simulink model "gm_uz_pmsm_model_9ph_vnl"  (R2021a)
settings: Solver=FixedStepAuto  StartTime=0.0  StopTime=.5  RelTol=1e-3
PreLoadFcn:
  | uz_pmsm_model_init_parameter
undefined symbols (not defined in the file or in its folder): c, friction_coefficient, inertia, k_i_d, k_p_d, k_p_q, L_d, L_o1, L_o2, L_q, L_x1, L_x2, L_y1, L_y2, L_zero, polepair, psi_pm, R_1, static_friction_torque, ts
libraries: hdlmdlgenlib x220, hdlsllib x18, simulink x11, pid_lib x2
(part 2 of 4)

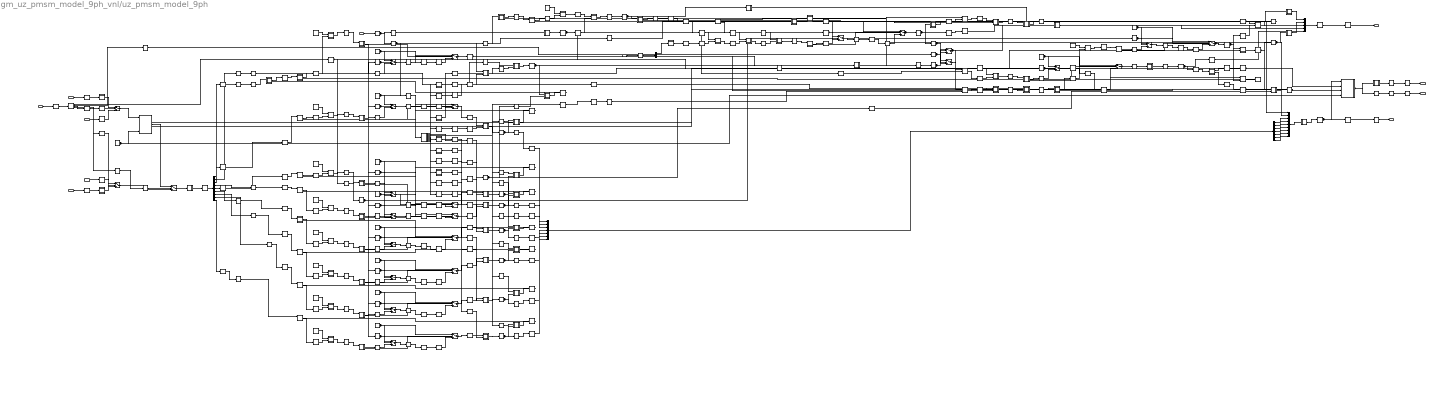
== system gm_uz_pmsm_model_9ph_vnl/uz_pmsm_model_9ph ==
  note: Input Processing
  note: o1 equation
  note: DQ equations
  note: o2 equation
  note: x1 equation
  note: y1 equation
  note: x2 equation
  note: y2 equation
  note: zero equation
  note: Output Processing
  Model_Parameter : Inport  SampleTime=1e-06
  Physical_Parameter : Inport  Port=2  SampleTime=1e-06
  inputs_general : Inport  Port=3  OutDataTypeStr=single  PortDimensions=[2]  SampleTime=1e-06
  input_voltages_dq : Inport  Port=4  OutDataTypeStr=single  PortDimensions=[9]  SampleTime=1e-06
  input_voltages_abc : Inport  Port=5  OutDataTypeStr=single  PortDimensions=[9]  SampleTime=1e-06
  u_dq_pl : Inport  Port=6  OutDataTypeStr=fixdt(1, 25, 12)  PortDimensions=[9]  SampleTime=1e-06
  u_abc_pl : Inport  Port=7  OutDataTypeStr=fixdt(1, 25, 12)  PortDimensions=[9]  SampleTime=1e-06
  Abs : Subsystem
      mask Display: disp('NFP\nabs');
  Abs_outbuff : hdlmdlgenlib/Buffer
      settings: SourceProductBaseCode=SL
  Add : Subsystem
      mask Display: disp('NFP\nadd');
  Add1 : Subsystem
      mask Display: disp('NFP\nadd');
  Add1_outbuff : hdlmdlgenlib/Buffer
      settings: SourceProductBaseCode=SL
  Add2 : Subsystem
      mask Display: disp('NFP\nadd');
  Add2_outbuff : hdlmdlgenlib/Buffer
      settings: SourceProductBaseCode=SL
  Add3 : Subsystem
      mask Display: disp('NFP\nadd');
  Add3_outbuff : hdlmdlgenlib/Buffer
      settings: SourceProductBaseCode=SL
  Add4 : Subsystem
      mask Display: disp('NFP\nadd');
  Add4_outbuff : hdlmdlgenlib/Buffer
      settings: SourceProductBaseCode=SL
  Add5 : Subsystem
      mask Display: disp('NFP\nadd');
  Add5_outbuff : hdlmdlgenlib/Buffer
      settings: SourceProductBaseCode=SL
  Add6 : Subsystem
      mask Display: disp('NFP\nadd');
  Add6_outbuff : hdlmdlgenlib/Buffer
      settings: SourceProductBaseCode=SL
  Add_outbuff : hdlmdlgenlib/Buffer
      settings: SourceProductBaseCode=SL
  Cos_to_sincos : Subsystem
      mask Display: disp('NFP\ntrig2');
  Cos_to_sincos_out1_buff : hdlmdlgenlib/Buffer
      settings: SourceProductBaseCode=SL
  Cos_to_sincos_out2_buff : hdlmdlgenlib/Buffer
      settings: SourceProductBaseCode=SL
  Data Type Conversion1 : Subsystem
      mask Display: disp('NFP\nconv');
  Data Type Conversion10 : Subsystem
      mask Display: disp('NFP\nconv');
  Data Type Conversion11 : Subsystem
      mask Display: disp('NFP\nconv');
  Data Type Conversion111 : Subsystem
      mask Display: disp('NFP\nconv');
  Data Type Conversion12 : Subsystem
      mask Display: disp('NFP\nconv');
  Data Type Conversion13 : Subsystem
      mask Display: disp('NFP\nconv');
  Data Type Conversion15 : Subsystem
      mask Display: disp('NFP\nconv');
  Data Type Conversion16 : Subsystem
      mask Display: disp('NFP\nconv');
  Data Type Conversion17 : Subsystem
      mask Display: disp('NFP\nconv');
  Data Type Conversion17_out1 : Delay  DelayLength=double(1)  InitialCondition=0  SampleTime=1e-08
  Data Type Conversion17_outbuff : hdlmdlgenlib/Buffer
      settings: SourceProductBaseCode=SL
  Data Type Conversion18 : Subsystem
      mask Display: disp('NFP\nconv');
  Data Type Conversion18_outbuff : hdlmdlgenlib/Buffer
      settings: SourceProductBaseCode=SL
  Data Type Conversion19 : Subsystem
      mask Display: disp('NFP\nconv');
  Data Type Conversion19_out1_0_wire : hdlmdlgenlib/Buffer
      settings: SourceProductBaseCode=SL
  Data Type Conversion19_out1_1_wire : hdlmdlgenlib/Buffer
      settings: SourceProductBaseCode=SL
  Data Type Conversion19_outbuff : hdlmdlgenlib/Buffer
      settings: SourceProductBaseCode=SL
  Data Type Conversion2 : Subsystem
      mask Display: disp('NFP\nconv');
  Data Type Conversion21 : Subsystem
      mask Display: disp('NFP\nconv');
  Data Type Conversion26 : Subsystem
      mask Display: disp('NFP\nconv');
  Data Type Conversion3 : Subsystem
      mask Display: disp('NFP\nconv');
  Data Type Conversion30 : Subsystem
      mask Display: disp('NFP\nconv');
  Data Type Conversion31 : Subsystem
      mask Display: disp('NFP\nconv');
  Data Type Conversion32 : Subsystem
      mask Display: disp('NFP\nconv');
  Data Type Conversion4 : Subsystem
      mask Display: disp('NFP\nconv');
  Data Type Conversion41 : Subsystem
      mask Display: disp('NFP\nconv');
  Data Type Conversion5 : Subsystem
      mask Display: disp('NFP\nconv');
  Data Type Conversion51 : Subsystem
      mask Display: disp('NFP\nconv');
  Data Type Conversion6 : Subsystem
      mask Display: disp('NFP\nconv');
  Data Type Conversion61 : Subsystem
      mask Display: disp('NFP\nconv');
  Data Type Conversion6_out1 : Delay  DelayLength=double(1)  InitialCondition=0  SampleTime=1e-08
  Data Type Conversion7 : DataTypeConversion  OutDataTypeStr=fixdt(1, 25, 12)  RndMeth=Nearest  SampleTime=1e-08
  Data Type Conversion71 : Subsystem
      mask Display: disp('NFP\nconv');
  Data Type Conversion7_out1 : Delay  DelayLength=double(1)  InitialCondition=0  SampleTime=1e-08
  Data Type Conversion8 : Subsystem
      mask Display: disp('NFP\nconv');
  Data Type Conversion9 : Subsystem
      mask Display: disp('NFP\nconv');
  Data Type Conversion91 : Subsystem
      mask Display: disp('NFP\nconv');
  Delay : RateTransition  OutPortSampleTimeOpt=Multiple of input port sample time  OutPortSampleTimeMultiple=100
  Delay1_lowered{,1..10} (11 alike) : RateTransition  OutPortSampleTimeOpt=Multiple of input port sample time  OutPortSampleTimeMultiple=100
  Delay1_toDel{,1..10} (11 alike) : Delay  DelayLength=double(1)  InitialCondition=0  SampleTime=1e-08
  Divide : Subsystem
      mask Display: disp('NFP\nmul');
  Divide1 : Subsystem
      mask Display: disp('NFP\nmul');
  Divide10 : Subsystem
      mask Display: disp('NFP\nmul');
  Divide10_outbuff : hdlmdlgenlib/Buffer
      settings: SourceProductBaseCode=SL
  Divide11 : Subsystem
      mask Display: disp('NFP\nmul');
  Divide11_outbuff : hdlmdlgenlib/Buffer
      settings: SourceProductBaseCode=SL
  Divide12 : Subsystem
      mask Display: disp('NFP\nmul');
  Divide12_outbuff : hdlmdlgenlib/Buffer
      settings: SourceProductBaseCode=SL
  Divide13 : Subsystem
      mask Display: disp('NFP\nmul');
  Divide13_outbuff : hdlmdlgenlib/Buffer
      settings: SourceProductBaseCode=SL
  Divide14 : Subsystem
      mask Display: disp('NFP\nmul');
  Divide1_outbuff : hdlmdlgenlib/Buffer
      settings: SourceProductBaseCode=SL
  Divide2 : Subsystem
      mask Display: disp('NFP\nmul');
  Divide2_outbuff : hdlmdlgenlib/Buffer
      settings: SourceProductBaseCode=SL
  Divide3 : Subsystem
      mask Display: disp('NFP\nmul');
  Divide3_outbuff : hdlmdlgenlib/Buffer
      settings: SourceProductBaseCode=SL
  Divide4 : Subsystem
      mask Display: disp('NFP\nmul');
  Divide4_outbuff : hdlmdlgenlib/Buffer
      settings: SourceProductBaseCode=SL
  Divide5 : Subsystem
      mask Display: disp('NFP\nmul');
  Divide5_outbuff : hdlmdlgenlib/Buffer
      settings: SourceProductBaseCode=SL
  Divide6 : Subsystem
      mask Display: disp('NFP\nmul');
  Divide6_outbuff : hdlmdlgenlib/Buffer
      settings: SourceProductBaseCode=SL
  Divide7 : Subsystem
      mask Display: disp('NFP\nmul');
  Divide7_outbuff : hdlmdlgenlib/Buffer
      settings: SourceProductBaseCode=SL
  Divide8 : Subsystem
      mask Display: disp('NFP\nmul');
  Divide8_outbuff : hdlmdlgenlib/Buffer
      settings: SourceProductBaseCode=SL
  Divide9 : Subsystem
      mask Display: disp('NFP\nmul');
  Divide9_outbuff : hdlmdlgenlib/Buffer
      settings: SourceProductBaseCode=SL
  Divide_outbuff : hdlmdlgenlib/Buffer
      settings: SourceProductBaseCode=SL
  Divide_outbuff1 : hdlmdlgenlib/Buffer
      settings: SourceProductBaseCode=SL
  Factor : Subsystem
      mask Display: disp('NFP\nmul');
  Factor_const : Constant  Value=double(4.5)  OutDataTypeStr=double  SampleTime=1e-08
  Factor_outbuff : hdlmdlgenlib/Buffer
      settings: SourceProductBaseCode=SL
  From{,1..34,40..52,61,71,81,91,101,110..111,121,131,161,210,461} (60 alike) : hdlmdlgenlib/Buffer
      settings: SourceProductBaseCode=SL
  Gain : Subsystem
      mask Display: disp('NFP\nmul');
  Gain1 : Subsystem
      mask Display: disp('NFP\nmul');
  Gain10 : Subsystem
      mask Display: disp('NFP\nmul');
  Gain2 : Subsystem
      mask Display: disp('NFP\nmul');
  Gain3 : Subsystem
      mask Display: disp('NFP\nmul');
  Gain4 : Subsystem
      mask Display: disp('NFP\nmul');
  Gain5 : Subsystem
      mask Display: disp('NFP\nmul');
  Gain6 : Subsystem
      mask Display: disp('NFP\nmul');
  Gain7 : Subsystem
      mask Display: disp('NFP\nmul');
  Gain8 : Subsystem
      mask Display: disp('NFP\nmul');
  Gain9 : Subsystem
      mask Display: disp('NFP\nmul');
  Gain_const{,1..10} (11 alike) : Constant  Value=double(1e-06)  OutDataTypeStr=double  SampleTime=1e-08
  Gain_outbuff{,1..10} (11 alike) : hdlmdlgenlib/Buffer
      settings: SourceProductBaseCode=SL
  Goto{,1..17,19,21..23,25,27,29..36,41,51,61,71,81,91,101,311} (40 alike) : hdlmdlgenlib/Buffer
      settings: SourceProductBaseCode=SL
  Initial_Val{,1..10} (11 alike) : Constant  Value=double(0)  OutDataTypeStr=double  SampleTime=1e-08
  M_Mi : hdlmdlgenlib/Buffer
      settings: SourceProductBaseCode=SL
  Mux_out1 : Delay  DelayLength=double(1)  InitialCondition=0  SampleTime=1e-08
  Product : Subsystem
      mask Display: disp('NFP\nmul');
  Product1 : Subsystem
      mask Display: disp('NFP\nmul');
  Product10 : Subsystem
      mask Display: disp('NFP\nmul');
  Product10_outbuff : hdlmdlgenlib/Buffer
      settings: SourceProductBaseCode=SL
  Product11 : Subsystem
      mask Display: disp('NFP\nmul');
  Product11_outbuff : hdlmdlgenlib/Buffer
      settings: SourceProductBaseCode=SL
  Product12 : Subsystem
      mask Display: disp('NFP\nmul');
  Product12_outbuff : hdlmdlgenlib/Buffer
      settings: SourceProductBaseCode=SL
  Product1_outbuff : hdlmdlgenlib/Buffer
      settings: SourceProductBaseCode=SL
  Product2 : Subsystem
      mask Display: disp('NFP\nmul');
  Product2_outbuff : hdlmdlgenlib/Buffer
      settings: SourceProductBaseCode=SL
  Product3 : Subsystem
      mask Display: disp('NFP\nmul');
  Product3_outbuff : hdlmdlgenlib/Buffer
      settings: SourceProductBaseCode=SL
  Product4 : Subsystem
      mask Display: disp('NFP\nmul');
  Product4_outbuff : hdlmdlgenlib/Buffer
      settings: SourceProductBaseCode=SL
  Product5 : Subsystem
      mask Display: disp('NFP\nmul');
  Product5_outbuff : hdlmdlgenlib/Buffer
      settings: SourceProductBaseCode=SL
  Product6 : Subsystem
      mask Display: disp('NFP\nmul');
  Product6_outbuff : hdlmdlgenlib/Buffer
      settings: SourceProductBaseCode=SL
  Product7 : Subsystem
      mask Display: disp('NFP\nmul');
  Product7_outbuff : hdlmdlgenlib/Buffer
      settings: SourceProductBaseCode=SL
  Product8 : Subsystem
      mask Display: disp('NFP\nmul');
  Product8_outbuff : hdlmdlgenlib/Buffer
      settings: SourceProductBaseCode=SL
  Product9 : Subsystem
      mask Display: disp('NFP\nmul');
  Product9_outbuff : hdlmdlgenlib/Buffer
      settings: SourceProductBaseCode=SL
  Product_outbuff : hdlmdlgenlib/Buffer
      settings: SourceProductBaseCode=SL
  Sign1 : Subsystem
      mask Display: disp('NFP\nsignum');
  Sign1_outbuff : hdlmdlgenlib/Buffer
      settings: SourceProductBaseCode=SL
  Sum : Subsystem
      mask Display: disp('NFP\nadd');
  Sum1 : Subsystem
      mask Display: disp('NFP\nadd');
  Sum1_outbuff : hdlmdlgenlib/Buffer
      settings: SourceProductBaseCode=SL
  Sum1_stage2 : Subsystem
      mask Display: disp('NFP\nadd');
  Sum1_stage2_outbuff : hdlmdlgenlib/Buffer
      settings: SourceProductBaseCode=SL
  Sum1_stage3 : Subsystem
      mask Display: disp('NFP\nadd');
  Sum1_stage3_outbuff : hdlmdlgenlib/Buffer
      settings: SourceProductBaseCode=SL
  Sum2 : Subsystem
      mask Display: disp('NFP\nadd');
  Sum2_outbuff : hdlmdlgenlib/Buffer
      settings: SourceProductBaseCode=SL
  Sum3 : Subsystem
      mask Display: disp('NFP\nadd');
  Sum31 : Subsystem
      mask Display: disp('NFP\nadd');
  Sum310 : Subsystem
      mask Display: disp('NFP\nadd');
  Sum311 : Subsystem
      mask Display: disp('NFP\nadd');
  Sum32 : Subsystem
      mask Display: disp('NFP\nadd');
  Sum33 : Subsystem
      mask Display: disp('NFP\nadd');
  Sum34 : Subsystem
      mask Display: disp('NFP\nadd');
  Sum35 : Subsystem
      mask Display: disp('NFP\nadd');
  Sum36 : Subsystem
      mask Display: disp('NFP\nadd');
  Sum37 : Subsystem
      mask Display: disp('NFP\nadd');
  Sum38 : Subsystem
      mask Display: disp('NFP\nadd');
  Sum39 : Subsystem
      mask Display: disp('NFP\nadd');
  Sum3_outbuff{,1..11} (12 alike) : hdlmdlgenlib/Buffer
      settings: SourceProductBaseCode=SL
  Sum5 : Subsystem
      mask Display: disp('NFP\nadd');
  Sum5_outbuff : hdlmdlgenlib/Buffer
      settings: SourceProductBaseCode=SL
  Sum_out1 : Delay  DelayLength=double(1)  InitialCondition=0  SampleTime=1e-08
  Sum_outbuff : hdlmdlgenlib/Buffer
      settings: SourceProductBaseCode=SL
  Sum_stage2 : Subsystem
      mask Display: disp('NFP\nadd');
  Sum_stage2_outbuff : hdlmdlgenlib/Buffer
      settings: SourceProductBaseCode=SL
  Sum_stage3 : Subsystem
      mask Display: disp('NFP\nadd');
  Sum_stage3_outbuff : hdlmdlgenlib/Buffer
      settings: SourceProductBaseCode=SL
  Switch : Switch  Criteria=u2 ~= 0  Threshold=double(0)  OutDataTypeStr=double  SampleTime=1e-08
  Switch1 : Switch  Criteria=u2 ~= 0  Threshold=double(0)  OutDataTypeStr=double  SampleTime=1e-08
  Switch2 : Switch  Criteria=u2 ~= 0  Threshold=double(0)  OutDataTypeStr=single  SampleTime=1e-08
  Switch3 : Switch  Criteria=u2 ~= 0  Threshold=double(0)  OutDataTypeStr=single  SampleTime=1e-08
  Switch4 : Switch  Criteria=u2 ~= 0  Threshold=double(0)  OutDataTypeStr=fixdt(1, 25, 12)  SampleTime=1e-08
  Transformation : Subsystem
  Transformation1 : Subsystem
  bus_selector : BusSelector  OutputSignals=1_L_d,1_L_q,R_1,polepair,psi_pm,L_o1,L_o2,L_x1,L_y1,L_x2,L_y2,L_zero
  bus_selector1 : BusSelector  OutputSignals=reset_integrators,simulate_mechanics,switch_pspl,control_dq_abc
  bus_selector2 : BusSelector  OutputSignals=polepair
  bus_selector3 : BusSelector  OutputSignals=mu,1_J,M_R0
  ctr_99 : simulink/Sources/Counter Limited  uplimit=double(99)  tsamp=1e-08
  i_d : hdlmdlgenlib/Buffer
      settings: SourceProductBaseCode=SL
  i_q : hdlmdlgenlib/Buffer
      settings: SourceProductBaseCode=SL
  in0_repeat : RateTransition  Integrity=off  Deterministic=off  OutPortSampleTimeOpt=Multiple of input port sample time  OutPortSampleTimeMultiple=1/100
  in10_repeat : RateTransition  Integrity=off  Deterministic=off  OutPortSampleTimeOpt=Multiple of input port sample time  OutPortSampleTimeMultiple=1/100
  in11_repeat : RateTransition  Integrity=off  Deterministic=off  OutPortSampleTimeOpt=Multiple of input port sample time  OutPortSampleTimeMultiple=1/100
  in12_repeat : RateTransition  Integrity=off  Deterministic=off  OutPortSampleTimeOpt=Multiple of input port sample time  OutPortSampleTimeMultiple=1/100
  in13_repeat : RateTransition  Integrity=off  Deterministic=off  OutPortSampleTimeOpt=Multiple of input port sample time  OutPortSampleTimeMultiple=1/100
  in14_repeat : RateTransition  Integrity=off  Deterministic=off  OutPortSampleTimeOpt=Multiple of input port sample time  OutPortSampleTimeMultiple=1/100
  in15_repeat : RateTransition  Integrity=off  Deterministic=off  OutPortSampleTimeOpt=Multiple of input port sample time  OutPortSampleTimeMultiple=1/100
  in16_repeat : RateTransition  Integrity=off  Deterministic=off  OutPortSampleTimeOpt=Multiple of input port sample time  OutPortSampleTimeMultiple=1/100
  in17_repeat : RateTransition  Integrity=off  Deterministic=off  OutPortSampleTimeOpt=Multiple of input port sample time  OutPortSampleTimeMultiple=1/100
  in18_repeat : RateTransition  Integrity=off  Deterministic=off  OutPortSampleTimeOpt=Multiple of input port sample time  OutPortSampleTimeMultiple=1/100
  in1_repeat : RateTransition  Integrity=off  Deterministic=off  OutPortSampleTimeOpt=Multiple of input port sample time  OutPortSampleTimeMultiple=1/100
  in2_repeat : RateTransition  Integrity=off  Deterministic=off  OutPortSampleTimeOpt=Multiple of input port sample time  OutPortSampleTimeMultiple=1/100
  in3_repeat : RateTransition  Integrity=off  Deterministic=off  OutPortSampleTimeOpt=Multiple of input port sample time  OutPortSampleTimeMultiple=1/100
  in4_repeat : RateTransition  Integrity=off  Deterministic=off  OutPortSampleTimeOpt=Multiple of input port sample time  OutPortSampleTimeMultiple=1/100
  in5_repeat : RateTransition  Integrity=off  Deterministic=off  OutPortSampleTimeOpt=Multiple of input port sample time  OutPortSampleTimeMultiple=1/100
  in6_repeat : RateTransition  Integrity=off  Deterministic=off  OutPortSampleTimeOpt=Multiple of input port sample time  OutPortSampleTimeMultiple=1/100
  in7_repeat : RateTransition  Integrity=off  Deterministic=off  OutPortSampleTimeOpt=Multiple of input port sample time  OutPortSampleTimeMultiple=1/100
  in8_repeat : RateTransition  Integrity=off  Deterministic=off  OutPortSampleTimeOpt=Multiple of input port sample time  OutPortSampleTimeMultiple=1/100
  in9_repeat : RateTransition  Integrity=off  Deterministic=off  OutPortSampleTimeOpt=Multiple of input port sample time  OutPortSampleTimeMultiple=1/100
  integrator1_out1 : hdlmdlgenlib/Buffer
      settings: SourceProductBaseCode=SL
  integrator1_out11 : hdlmdlgenlib/Buffer
      settings: SourceProductBaseCode=SL
  mechanical_system_out1 : hdlmdlgenlib/Buffer
      settings: SourceProductBaseCode=SL
  mux : Mux  Inputs=7
  mux1 : Mux  Inputs=9
  mux2 : Mux  Inputs=5
  pmsm_out3 : hdlmdlgenlib/Buffer
      settings: SourceProductBaseCode=SL
  pmsm_out4 : hdlmdlgenlib/Buffer
      settings: SourceProductBaseCode=SL
  psi_{,1..6} (7 alike) : hdlmdlgenlib/Buffer
      settings: SourceProductBaseCode=SL
  psi_d : hdlmdlgenlib/Buffer
      settings: SourceProductBaseCode=SL
  psi_q : hdlmdlgenlib/Buffer
      settings: SourceProductBaseCode=SL
  reset_in{,1..10} (11 alike) : Switch  Criteria=u2 ~= 0  Threshold=double(0)  OutDataTypeStr=double  SampleTime=1e-08
  reset_out{,1..10} (11 alike) : Switch  Criteria=u2 ~= 0  Threshold=double(0)  OutDataTypeStr=double  SampleTime=1e-08
  t : Demux  Outputs=2
  t1 : Demux  Outputs=9
  t2 : Demux  Outputs=7
  t{3..6} (4 alike) : RateTransition  OutPortSampleTimeOpt=Multiple of input port sample time  OutPortSampleTimeMultiple=100
  output_general : Outport  SampleTime=1e-06
  output_currents_dq : Outport  Port=2  SampleTime=1e-06
  output_currents_abc : Outport  Port=3  SampleTime=1e-06
  u_abc_pl_out : Outport  Port=4  SampleTime=1e-06
  wires:
  ctr_99/1 -> Transformation/4(enb_counter), Transformation1/4(enb_counter)
  Gain10/1(Out1) -> Gain_outbuff10/1
  Factor/1(Out1) -> Factor_outbuff/1
  Gain9/1(Out1) -> Gain_outbuff9/1
  Gain8/1(Out1) -> Gain_outbuff8/1
  Gain7/1(Out1) -> Gain_outbuff7/1
  Gain6/1(Out1) -> Gain_outbuff6/1
  Gain5/1(Out1) -> Gain_outbuff5/1
  Gain4/1(Out1) -> Gain_outbuff4/1
  Gain3/1(Out1) -> Gain_outbuff3/1
  Gain2/1(Out1) -> Gain_outbuff2/1
  Gain1/1(Out1) -> Gain_outbuff1/1
  Gain/1(Out1) -> Gain_outbuff/1
  Cos_to_sincos/2(Out2) -> Cos_to_sincos_out2_buff/1
  Cos_to_sincos/1(Out1) -> Cos_to_sincos_out1_buff/1
  Data Type Conversion91/1(Out1) -> Product12/1(In1)
  Product12/1(Out1) -> Product12_outbuff/1
  Sum5/1(Out1) -> Sum5_outbuff/1
  Data Type Conversion13/1(Out1) -> Sum5/2(In2)
  Product4/1(Out1) -> Product4_outbuff/1
  Sum/1(Out1) -> Sum_outbuff/1
  Data Type Conversion15/1(Out1) -> mux2/3
  Data Type Conversion26/1(Out1) -> mux2/1
  Data Type Conversion17/1(Out1) -> Data Type Conversion17_outbuff/1
  Data Type Conversion19/1(Out1) -> Data Type Conversion19_outbuff/1
  Sum_stage3/1(Out1) -> Sum_stage3_outbuff/1
  Sum_stage2/1(Out1) -> Sum_stage2_outbuff/1
  Sum311/1(Out1) -> Sum3_outbuff11/1
  Product3/1(Out1) -> Product3_outbuff/1
  Sum310/1(Out1) -> Sum3_outbuff10/1
  Product9/1(Out1) -> Product9_outbuff/1
  Data Type Conversion32/1(Out1) -> Goto/1
  Divide14/1(Out1) -> Divide_outbuff1/1
  Sum39/1(Out1) -> Sum3_outbuff9/1
  Abs/1(Out1) -> Abs_outbuff/1
  Sign1/1(Out1) -> Sign1_outbuff/1
  Data Type Conversion30/1(Out1) -> Switch2/3
  Data Type Conversion31/1(Out1) -> Switch4/1
  Data Type Conversion41/1(Out1) -> Goto16/1
  Data Type Conversion51/1(Out1) -> Goto22/1
  Sum1/1(Out1) -> Sum1_outbuff/1
  Product11/1(Out1) -> Product11_outbuff/1
  Data Type Conversion21/1(Out1) -> Product11/1(In1)
  Sum38/1(Out1) -> Sum3_outbuff8/1
  Data Type Conversion16/1(Out1) -> mux2/4
  Product10/1(Out1) -> Product10_outbuff/1
  Product1/1(Out1) -> Product1_outbuff/1
  Sum1_stage3/1(Out1) -> Sum1_stage3_outbuff/1
  Sum1_stage2/1(Out1) -> Sum1_stage2_outbuff/1
  Sum37/1(Out1) -> Sum3_outbuff7/1
  Product/1(Out1) -> Product_outbuff/1
  Product6/1(Out1) -> Product6_outbuff/1
  Product7/1(Out1) -> Product7_outbuff/1
  Divide2/1(Out1) -> Divide2_outbuff/1
  Add1/1(Out1) -> Add1_outbuff/1
  Sum36/1(Out1) -> Sum3_outbuff6/1
  Divide3/1(Out1) -> Divide3_outbuff/1
  Divide1/1(Out1) -> Divide1_outbuff/1
  Divide/1(Out1) -> Divide_outbuff/1
  Add/1(Out1) -> Add_outbuff/1
  Sum35/1(Out1) -> Sum3_outbuff5/1
  Divide13/1(Out1) -> Divide13_outbuff/1
  Data Type Conversion61/1(Out1) -> Goto15/1
  Data Type Conversion5/1(Out1) -> Goto14/1
  Divide11/1(Out1) -> Divide11_outbuff/1
  Divide10/1(Out1) -> Divide10_outbuff/1
  Add5/1(Out1) -> Add5_outbuff/1
  Sum34/1(Out1) -> Sum3_outbuff4/1
  Data Type Conversion4/1(Out1) -> Goto13/1
  Divide9/1(Out1) -> Divide9_outbuff/1
  Divide8/1(Out1) -> Divide8_outbuff/1
  Add4/1(Out1) -> Add4_outbuff/1
  Sum33/1(Out1) -> Sum3_outbuff3/1
  Data Type Conversion3/1(Out1) -> Goto12/1
  Divide7/1(Out1) -> Divide7_outbuff/1
  Divide6/1(Out1) -> Divide6_outbuff/1
  Add3/1(Out1) -> Add3_outbuff/1
  Sum32/1(Out1) -> Sum3_outbuff2/1
  Data Type Conversion2/1(Out1) -> Goto11/1
  Divide5/1(Out1) -> Divide5_outbuff/1
  Divide4/1(Out1) -> Divide4_outbuff/1
  Add2/1(Out1) -> Add2_outbuff/1
  Sum31/1(Out1) -> Sum3_outbuff1/1
  Data Type Conversion1/1(Out1) -> Goto10/1
  Data Type Conversion10/1(Out1) -> Goto9/1
  Data Type Conversion8/1(Out1) -> Goto34/1
  Data Type Conversion71/1(Out1) -> Goto32/1
  Data Type Conversion12/1(Out1) -> Goto35/1
  Data Type Conversion111/1(Out1) -> Goto36/1
  Product5/1(Out1) -> Product5_outbuff/1
  Sum2/1(Out1) -> Sum2_outbuff/1
  Data Type Conversion9/1(Out1) -> Goto33/1
  Product8/1(Out1) -> Product8_outbuff/1
  Divide12/1(Out1) -> Divide12_outbuff/1
  Add6/1(Out1) -> Add6_outbuff/1
  Sum3/1(Out1) -> Sum3_outbuff/1
  Data Type Conversion11/1(Out1) -> mux2/2
  Product2/1(Out1) -> Product2_outbuff/1
  Data Type Conversion18/1(Out1) -> Data Type Conversion18_outbuff/1
  Data Type Conversion6/1(Out1) -> Data Type Conversion6_out1/1
  reset_in4/1 -> Delay1_toDel8/1
  reset_in3/1 -> Delay1_toDel7/1
  reset_in2/1 -> Delay1_toDel6/1
  reset_in1/1 -> Delay1_toDel5/1
  reset_in/1 -> Delay1_toDel4/1
  reset_in5/1 -> Delay1_toDel3/1
  reset_in6/1 -> Delay1_toDel2/1
  reset_in7/1 -> Delay1_toDel1/1
  reset_in10/1 -> Delay1_toDel/1
  Data Type Conversion7/1 -> Data Type Conversion7_out1/1
  Data Type Conversion17_outbuff/1 -> Data Type Conversion17_out1/1, Transformation1/1(in)
  reset_in8/1 -> Delay1_toDel10/1
  reset_in9/1 -> Delay1_toDel9/1
  mux2/1 -> Mux_out1/1
  Sum_outbuff/1 -> Sum_out1/1
  From27/1 -> reset_in4/2, reset_out3/2
  reset_out3/1 -> Sum34/2(In2), psi_4/1
  Divide10_outbuff/1 -> Add5/2(In2)
  From23/1 -> reset_in3/2, reset_out2/2
  reset_out2/1 -> Sum33/2(In2), psi_3/1
  Divide8_outbuff/1 -> Add4/2(In2)
  From19/1 -> reset_in2/2, reset_out1/2
  reset_out1/1 -> Sum32/2(In2), psi_2/1
  Divide6_outbuff/1 -> Add3/2(In2)
  From15/1 -> reset_in1/2, reset_out/2
  reset_out/1 -> Sum31/2(In2), psi_1/1
  Divide4_outbuff/1 -> Add2/2(In2)
  From31/1 -> reset_in/2, reset_out4/2
  reset_out4/1 -> Sum3/2(In2), psi_5/1
  Divide12_outbuff/1 -> Add6/2(In2)
  From5/1 -> reset_in5/2, reset_out5/2
  reset_out5/1 -> Sum35/2(In2), psi_/1
  Divide_outbuff/1 -> Add/2(In2)
  From9/1 -> reset_in6/2, reset_out6/2
  reset_out6/1 -> Sum36/2(In2), psi_6/1
  Divide2_outbuff/1 -> Add1/2(In2)
  From3/1 -> reset_in7/2, reset_out7/2
  reset_out7/1 -> Sum37/2(In2), psi_q/1
  Product7_outbuff/1 -> Sum1_stage3/2(In2)
  Product1_outbuff/1 -> Sum1_stage2/2(In2)
  From2/1 -> reset_in10/2, reset_out10/2
  reset_out10/1 -> Sum311/2(In2), psi_d/1
  Product_outbuff/1 -> Sum_stage3/2(In2)
  Product8_outbuff/1 -> Sum_stage2/2(In2)
  Switch2/1 -> Switch3/3
  From121/1 -> Switch3/2
  Gain_const10/1 -> Gain10/1(In1)
  Factor_const/1 -> Factor/1(In1)
  Gain_const9/1 -> Gain9/1(In1)
  Gain_const8/1 -> Gain8/1(In1)
  Gain_const7/1 -> Gain7/1(In1)
  Gain_const6/1 -> Gain6/1(In1)
  Gain_const5/1 -> Gain5/1(In1)
  Gain_const4/1 -> Gain4/1(In1)
  Gain_const3/1 -> Gain3/1(In1)
  Gain_const2/1 -> Gain2/1(In1)
  Gain_const1/1 -> Gain1/1(In1)
  Gain_const/1 -> Gain/1(In1)
  t2/7 -> mux1/9
  t2/6 -> mux1/8
  t2/5 -> mux1/7
  t2/4 -> mux1/6
  t2/3 -> mux1/5
  t2/2 -> mux1/4
  t2/1 -> mux1/3
  t1/9 -> Goto81/1
  t1/8 -> Goto7/1
  t1/7 -> Goto6/1
  t1/6 -> Goto51/1
  t1/5 -> Goto4/1
  t1/4 -> Goto3/1
  t1/3 -> Goto2/1
  t1/2 -> Data Type Conversion19_out1_1_wire/1
  t1/1 -> Data Type Conversion19_out1_0_wire/1
  Sum_stage2_outbuff/1 -> Sum_stage3/1(In1)
  t/2 -> Data Type Conversion41/1(In1)
  t/1 -> Data Type Conversion51/1(In1)
  Sum1_stage2_outbuff/1 -> Sum1_stage3/1(In1)
  bus_selector3/3 -> Data Type Conversion21/1(In1)  "<M_R0>"
  bus_selector3/2 -> Data Type Conversion13/1(In1)  "<1_J>"
  bus_selector3/1 -> Data Type Conversion91/1(In1)  "<mu>"
  Product12_outbuff/1 -> Sum5/1(In1)
  Sum5_outbuff/1 -> Product4/1(In1)
  Product4_outbuff/1 -> Sum/2(In2)
  M_Mi/1 -> Data Type Conversion15/1(In1), Sum/1(In1)
  i_d/1 -> mux1/1, Product2/1(In1), Data Type Conversion26/1(In1)
  mux1/1 -> Data Type Conversion17/1(In1)
  Transformation1/1(out) -> Data Type Conversion7/1, Data Type Conversion6/1(In1)
  Goto61/1 -> Transformation/2(sin_theta_el), Transformation1/2(sin_theta_el)
  Transformation/1(out) -> Switch3/1
  Switch3/1 -> Data Type Conversion19/1(In1)
  Data Type Conversion19_outbuff/1 -> t1/1
  Data Type Conversion19_out1_1_wire/1 -> Goto30/1
  Data Type Conversion19_out1_0_wire/1 -> Goto311/1
  Goto311/1 -> From461/1
  From461/1 -> Sum_stage2/1(In1)
  Sum_stage3_outbuff/1 -> Gain10/2(In2)
  Gain_outbuff10/1 -> Sum311/1(In1)
  Sum3_outbuff11/1 -> reset_in10/3
  Initial_Val10/1 -> reset_in10/1, reset_out10/1
  psi_d/1 -> pmsm_out3/1, Sum2/1(In1), Product1/2(In2)
  pmsm_out3/1 -> Product3/1(In1)
  Product3_outbuff/1 -> Sum310/1(In1)
  Sum3_outbuff10/1 -> Factor/2(In2)
  Factor_outbuff/1 -> Product9/1(In1)
  Product9_outbuff/1 -> M_Mi/1
  From34/1 -> Product9/2(In2)
  Goto/1 -> From34/1, From71/1
  bus_selector2/1 -> Data Type Conversion32/1(In1)  "<polepair>"
  From71/1 -> Divide14/2(In2)
  Divide_outbuff1/1 -> Gain9/2(In2)
  Gain_outbuff9/1 -> Sum39/1(In1)
  Sum3_outbuff9/1 -> reset_in9/3
  Initial_Val9/1 -> reset_in9/1, reset_out9/1
  reset_out9/1 -> integrator1_out1/1, Sum39/2(In2)
  From61/1 -> reset_in9/2, reset_out9/2
  Goto31/1 -> From32/1, From46/1, From61/1
  From46/1 -> reset_in8/2, reset_out8/2
  reset_out8/1 -> integrator1_out11/1, Sum38/2(In2)
  integrator1_out11/1 -> mechanical_system_out1/1, Sign1/1(In1), Abs/1(In1)
  Abs_outbuff/1 -> Product12/2(In2)
  Sign1_outbuff/1 -> Product4/2(In2)
  mechanical_system_out1/1 -> Switch1/1, Switch/1
  Switch/1 -> Product10/1(In1)
  From52/1 -> Switch1/2, Switch/2
  Goto41/1 -> From52/1
  bus_selector1/4 -> Goto101/1  "<control_dq_abc>"
  bus_selector1/3 -> Goto91/1  "<switch_pspl>"
  bus_selector1/2 -> Goto41/1  "<simulate_mechanics>"
  bus_selector1/1 -> Goto31/1  "<reset_integrators>"
  Goto101/1 -> From121/1
  Goto91/1 -> From111/1, From131/1
  From111/1 -> Switch2/2
  From131/1 -> Switch4/2
  Switch4/1 -> Transformation/1(in)
  Switch1/1 -> Data Type Conversion16/1(In1), Divide14/1(In1)
  From210/1 -> Switch1/3, Switch/3
  Goto16/1 -> From210/1
  Goto22/1 -> From110/1
  From110/1 -> Sum1/2(In2)
  Sum1_outbuff/1 -> Product11/2(In2)
  Product11_outbuff/1 -> Gain8/2(In2)
  Gain_outbuff8/1 -> Sum38/1(In1)
  Sum3_outbuff8/1 -> reset_in8/3
  Initial_Val8/1 -> reset_in8/1, reset_out8/1
  Product10_outbuff/1 -> Product/1(In1), Product1/1(In1)
  Sum1_stage3_outbuff/1 -> Gain7/2(In2)
  From47/1 -> Sum1_stage2/1(In1)
  Goto30/1 -> From47/1
  Gain_outbuff7/1 -> Sum37/1(In1)
  Sum3_outbuff7/1 -> reset_in7/3
  Initial_Val7/1 -> reset_in7/1, reset_out7/1
  psi_q/1 -> pmsm_out4/1, Product6/1(In1), Product/2(In2)
  Product6_outbuff/1 -> i_q/1, Product7/1(In1)
  From1/1 -> Product7/2(In2)
  Goto32/1 -> From/1, From1/1, From14/1, From18/1, From22/1, From26/1, From30/1, From4/1, From81/1
  From81/1 -> Divide2/1(In1)
  Add1_outbuff/1 -> Gain6/2(In2)
  From101/1 -> Add1/1(In1)
  Goto3/1 -> From101/1
  Gain_outbuff6/1 -> Sum36/1(In1)
  Sum3_outbuff6/1 -> reset_in6/3
  Initial_Val6/1 -> reset_in6/1, reset_out6/1
  psi_6/1 -> Divide3/1(In1)
  Divide3_outbuff/1 -> Goto19/1, Divide2/2(In2)
  Goto19/1 -> From40/1
  From40/1 -> mux/2
  mux/1 -> t2/1
  From33/1 -> mux/1
  Goto17/1 -> From33/1
  Divide1_outbuff/1 -> Goto17/1, Divide/2(In2)
  From4/1 -> Divide/1(In1)
  Add_outbuff/1 -> Gain5/2(In2)
  From6/1 -> Add/1(In1)
  Goto2/1 -> From6/1
  Gain_outbuff5/1 -> Sum35/1(In1)
  Sum3_outbuff5/1 -> reset_in5/3
  Initial_Val5/1 -> reset_in5/1, reset_out5/1
  Goto1/1 -> From15/1, From19/1, From2/1, From23/1, From27/1, From3/1, From31/1, From5/1, From9/1
  From32/1 -> Goto1/1
  psi_5/1 -> Divide13/1(In1)
  Divide13_outbuff/1 -> Goto29/1, Divide12/2(In2)
  From29/1 -> Divide13/2(In2)
  Goto15/1 -> From29/1
  bus_selector/12 -> Data Type Conversion61/1(In1)  "<L_zero>"
  bus_selector/11 -> Data Type Conversion5/1(In1)  "<L_y2>"
  bus_selector/10 -> Data Type Conversion4/1(In1)  "<L_x2>"
  bus_selector/9 -> Data Type Conversion3/1(In1)  "<L_y1>"
  bus_selector/8 -> Data Type Conversion2/1(In1)  "<L_x1>"
  bus_selector/7 -> Data Type Conversion1/1(In1)  "<L_o2>"
  bus_selector/6 -> Data Type Conversion10/1(In1)  "<L_o1>"
  bus_selector/5 -> Data Type Conversion9/1(In1)  "<psi_pm>"
  bus_selector/4 -> Data Type Conversion8/1(In1)  "<polepair>"
  bus_selector/3 -> Data Type Conversion71/1(In1)  "<R_1>"
  bus_selector/2 -> Data Type Conversion12/1(In1)  "<1_L_q>"
  bus_selector/1 -> Data Type Conversion111/1(In1)  "<1_L_d>"
  From8/1 -> bus_selector/1
  Goto71/1 -> From8/1, From91/1
  From91/1 -> bus_selector3/1
  Goto14/1 -> From25/1
  From25/1 -> Divide11/2(In2)
  Divide11_outbuff/1 -> Goto27/1, Divide10/2(In2)
  From26/1 -> Divide10/1(In1)
  Add5_outbuff/1 -> Gain4/2(In2)
  From24/1 -> Add5/1(In1)
  Goto7/1 -> From24/1
  Gain_outbuff4/1 -> Sum34/1(In1)
  Sum3_outbuff4/1 -> reset_in4/3
  Initial_Val4/1 -> reset_in4/1, reset_out3/1
  psi_4/1 -> Divide11/1(In1)
  Goto27/1 -> From44/1
  From44/1 -> mux/6
  Goto13/1 -> From21/1
  From21/1 -> Divide9/2(In2)
  Divide9_outbuff/1 -> Goto25/1, Divide8/2(In2)
  From22/1 -> Divide8/1(In1)
  Add4_outbuff/1 -> Gain3/2(In2)
  From20/1 -> Add4/1(In1)
  Goto6/1 -> From20/1
  Gain_outbuff3/1 -> Sum33/1(In1)
  Sum3_outbuff3/1 -> reset_in3/3
  Initial_Val3/1 -> reset_in3/1, reset_out2/1
  psi_3/1 -> Divide9/1(In1)
  Goto25/1 -> From43/1
  From43/1 -> mux/5
  Goto12/1 -> From17/1
  From17/1 -> Divide7/2(In2)
  Divide7_outbuff/1 -> Goto23/1, Divide6/2(In2)
  From18/1 -> Divide6/1(In1)
  Add3_outbuff/1 -> Gain2/2(In2)
  From161/1 -> Add3/1(In1)
  Goto51/1 -> From161/1
  Gain_outbuff2/1 -> Sum32/1(In1)
  Sum3_outbuff2/1 -> reset_in2/3
  Initial_Val2/1 -> reset_in2/1, reset_out1/1
  psi_2/1 -> Divide7/1(In1)
  Goto23/1 -> From42/1
  From42/1 -> mux/4
  Goto11/1 -> From13/1
  From13/1 -> Divide5/2(In2)
  Divide5_outbuff/1 -> Goto21/1, Divide4/2(In2)
  From14/1 -> Divide4/1(In1)
  Add2_outbuff/1 -> Gain1/2(In2)
  From12/1 -> Add2/1(In1)
  Goto4/1 -> From12/1
  Gain_outbuff1/1 -> Sum31/1(In1)
  Sum3_outbuff1/1 -> reset_in1/3
  Initial_Val1/1 -> reset_in1/1, reset_out/1
  psi_1/1 -> Divide5/1(In1)
  Goto21/1 -> From41/1
  From41/1 -> mux/3
  Goto10/1 -> From11/1
  From11/1 -> Divide3/2(In2)
  Goto9/1 -> From7/1
  From7/1 -> Divide1/2(In2)
  Goto34/1 -> From49/1
  From49/1 -> Product10/2(In2)
  Goto35/1 -> From51/1
  From51/1 -> Product6/2(In2)
  Goto36/1 -> From50/1
  From50/1 -> Product5/1(In1)
  Product5_outbuff/1 -> i_d/1, Product8/1(In1)
  Sum2_outbuff/1 -> Product5/2(In2)
  From48/1 -> Sum2/2(In2)
  Goto33/1 -> From48/1
  From/1 -> Product8/2(In2)
  From30/1 -> Divide12/1(In1)
  Add6_outbuff/1 -> Gain/2(In2)
  From28/1 -> Add6/1(In1)
  Goto81/1 -> From28/1
  Gain_outbuff/1 -> Sum3/1(In1)
  Sum3_outbuff/1 -> reset_in/3
  Initial_Val/1 -> reset_in/1, reset_out4/1
  Goto29/1 -> From45/1
  From45/1 -> mux/7
  psi_/1 -> Divide1/1(In1)
  i_q/1 -> mux1/2, Data Type Conversion11/1(In1), Product3/2(In2)
  pmsm_out4/1 -> Product2/2(In2)
  Product2_outbuff/1 -> Sum310/2(In2)
  integrator1_out1/1 -> Data Type Conversion18/1(In1)
  Data Type Conversion18_outbuff/1 -> Goto5/1
  Goto5/1 -> From10/1, From16/1
  From10/1 -> mux2/5
  From16/1 -> Cos_to_sincos/1(In1)
  Cos_to_sincos_out1_buff/1 -> Goto61/1
  Cos_to_sincos_out2_buff/1 -> Goto8/1
  Goto8/1 -> Transformation/3(cos_theta_el), Transformation1/3(cos_theta_el)
  in18_repeat/1 -> reset_out10/3
  in17_repeat/1 -> reset_out9/3
  in16_repeat/1 -> reset_out8/3
  in15_repeat/1 -> bus_selector1/1
  in14_repeat/1 -> Data Type Conversion30/1(In1)
  in13_repeat/1 -> Switch2/1
  in12_repeat/1 -> Switch4/3
  in11_repeat/1 -> Data Type Conversion31/1(In1)
  in10_repeat/1 -> t/1
  in9_repeat/1 -> Sum1/1(In1)
  in8_repeat/1 -> reset_out7/3
  in7_repeat/1 -> reset_out6/3
  in6_repeat/1 -> reset_out5/3
  in5_repeat/1 -> reset_out4/3
  in4_repeat/1 -> Goto71/1, bus_selector2/1
  in3_repeat/1 -> reset_out3/3
  in2_repeat/1 -> reset_out2/3
  in1_repeat/1 -> reset_out1/3
  in0_repeat/1 -> reset_out/3
  Data Type Conversion17_out1/1 -> t6/1
  Delay1_toDel10/1 -> Delay1_lowered10/1
  Delay1_toDel8/1 -> Delay1_lowered9/1
  Delay1_toDel7/1 -> Delay1_lowered8/1
  Delay1_toDel6/1 -> Delay1_lowered7/1
  Delay1_toDel5/1 -> Delay1_lowered6/1
  Delay1_toDel4/1 -> Delay1_lowered5/1
  Delay1_toDel3/1 -> Delay1_lowered4/1
  Delay1_toDel2/1 -> Delay1_lowered3/1
  Delay1_toDel1/1 -> Delay1_lowered2/1
  Delay1_toDel9/1 -> Delay1_lowered1/1
  Delay1_toDel/1 -> Delay1_lowered/1
  Data Type Conversion6_out1/1 -> t5/1
  Data Type Conversion7_out1/1 -> t4/1
  Mux_out1/1 -> t3/1
  Sum_out1/1 -> Delay/1
  Delay1_lowered10/1 -> in16_repeat/1
  Delay1_lowered9/1 -> in3_repeat/1
  Delay1_lowered8/1 -> in2_repeat/1
  Delay1_lowered7/1 -> in1_repeat/1
  Delay1_lowered6/1 -> in0_repeat/1
  Delay1_lowered5/1 -> in5_repeat/1
  Delay1_lowered4/1 -> in6_repeat/1
  Delay1_lowered3/1 -> in7_repeat/1
  Delay1_lowered2/1 -> in8_repeat/1
  Delay1_lowered1/1 -> in17_repeat/1
  Delay1_lowered/1 -> in18_repeat/1
  Delay/1 -> in9_repeat/1
  t6/1 -> output_currents_dq/1
  t5/1 -> output_currents_abc/1
  t4/1 -> u_abc_pl_out/1
  t3/1 -> output_general/1
  u_abc_pl/1 -> in12_repeat/1
  u_dq_pl/1 -> in14_repeat/1
  input_voltages_abc/1 -> in11_repeat/1
  input_voltages_dq/1 -> in13_repeat/1
  inputs_general/1 -> in10_repeat/1
  Physical_Parameter/1 -> in4_repeat/1
  Model_Parameter/1 -> in15_repeat/1

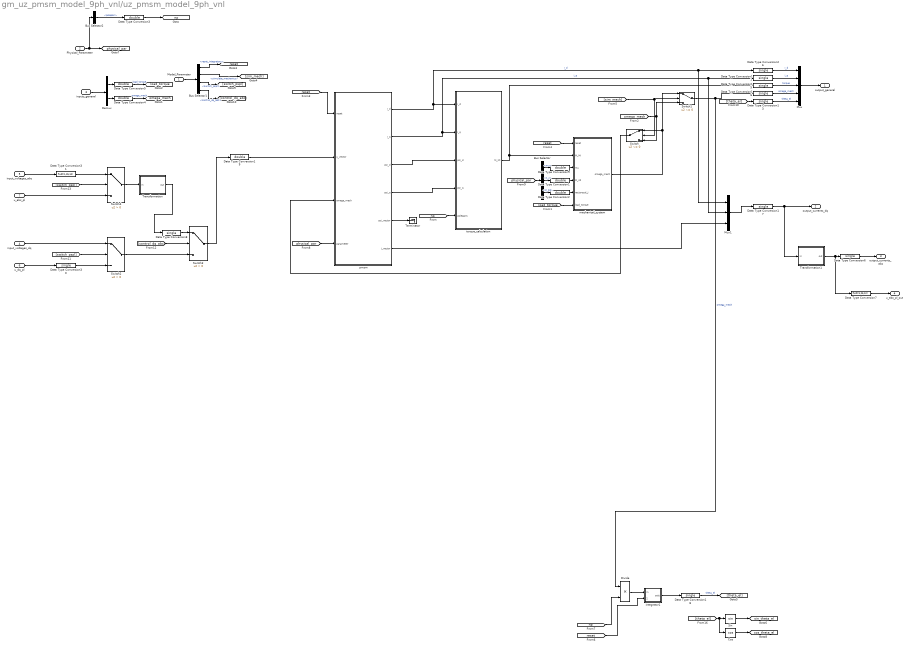
== system gm_uz_pmsm_model_9ph_vnl/uz_pmsm_model_9ph_vnl ==
  Model_Parameter : Inport
  Physical_Parameter : Inport  Port=2
  inputs_general : Inport  Port=3
  input_voltages_dq : Inport  Port=4
  input_voltages_abc : Inport  Port=5
  u_dq_pl : Inport  Port=6
  u_abc_pl : Inport  Port=7
  Bus Selector : BusSelector  OutputSignals=mu,1_J,M_R0
  Bus Selector1 : BusSelector  OutputSignals=reset_integrators,simulate_mechanics,switch_pspl,control_dq_abc
  Bus Selector2 : BusSelector  OutputSignals=polepair
  Cos : Trigonometry  Operator=cos
  Data Type Conversion{1..5,9,19} (7 alike) : DataTypeConversion  OutDataTypeStr=double  RndMeth=Nearest
  Data Type Conversion{6,8,11,13,15..18,26,30} (10 alike) : DataTypeConversion  OutDataTypeStr=single  RndMeth=Nearest
  Data Type Conversion31 : DataTypeConversion  OutDataTypeStr=fixdt(1,25,12)  RndMeth=Nearest
  Data Type Conversion7 : DataTypeConversion  OutDataTypeStr=fixdt(1,25,12)  RndMeth=Nearest
  Demux : Demux  Outputs=2
  Divide : Product  Inputs=**
  Mux : Mux  Inputs=5
  Mux1 : Mux  Inputs=3
  Sin : Trigonometry
  Switch : Switch  Criteria=u2 ~= 0
  Switch1 : Switch  Criteria=u2 ~= 0
  Switch2 : Switch  Criteria=u2 > Threshold
  Switch3 : Switch  Criteria=u2 > Threshold
  Switch4 : Switch  Criteria=u2 > Threshold
  Terminator : Terminator
  Transformation : Subsystem
  Transformation1 : Subsystem
  integrator1 : Subsystem
  mechanical_system : Subsystem
  pmsm : Subsystem
  torque_calculation : Subsystem
  output_general : Outport
  output_currents_dq : Outport  Port=2
  output_currents_abc : Outport  Port=3
  u_abc_pl_out : Outport  Port=4
  tag scope: cos_theta_el=global, load_torque=global, np=global, omega_mech=global, physical_par=global, reset=global, sin_theta_el=global
  wires:
  Transformation/1(out) -> Data Type Conversion8/1
  Data Type Conversion8/1 -> Switch3/1
  Data Type Conversion7/1 -> u_abc_pl_out/1
  Data Type Conversion6/1 -> output_currents_abc/1
  Mux1/1 -> Data Type Conversion17/1
  pmsm/6(I_vector) -> Mux1/3
  Switch4/1 -> Transformation/1(in)
  [switch_pspl] -> Switch4/2
  Data Type Conversion31/1 -> Switch4/1
  Switch3/1 -> Data Type Conversion19/1
  [control_dq_abc] -> Switch3/2
  Switch2/1 -> Switch3/3
  Data Type Conversion30/1 -> Switch2/3
  [switch_pspl] -> Switch2/2
  [theta_el] -> Data Type Conversion13/1
  Demux/1 -> Data Type Conversion5/1
  Demux/2 -> Data Type Conversion4/1
  Data Type Conversion3/1 -> [np]
  Bus Selector2/1 -> Data Type Conversion3/1  "<polepair>"
  Bus Selector/3 -> Data Type Conversion2/1  "<M_R0>"
  Bus Selector/2 -> Data Type Conversion1/1  "<1_J>"
  Bus Selector/1 -> Data Type Conversion9/1  "<mu>"
  Data Type Conversion2/1 -> mechanical_system/5(reciprocal_J)
  Data Type Conversion1/1 -> mechanical_system/4(M_n0)
  Data Type Conversion9/1 -> mechanical_system/3(mu)
  [physical_par] -> Bus Selector/1
  [physical_par] -> pmsm/4(parameter)
  Physical_Parameter/1 -> [physical_par], Bus Selector2/1
  Data Type Conversion19/1 -> pmsm/2(u_vector)
  u_abc_pl/1 -> Switch4/3
  u_dq_pl/1 -> Data Type Conversion30/1
  [np] -> Divide/2
  Switch1/1 -> Data Type Conversion16/1, Divide/1  "omega_mech"
  Divide/1 -> integrator1/1(in)
  Sin/1 -> [sin_theta_el]
  Data Type Conversion18/1 -> [theta_el]  "theta_el"
  [reset] -> integrator1/2(reset)
  integrator1/1(outt) -> Data Type Conversion18/1
  [theta_el] -> Sin/1, Cos/1
  Cos/1 -> [cos_theta_el]
  Data Type Conversion17/1 -> output_currents_dq/1, Transformation1/1(in)
  Transformation1/1(out) -> Data Type Conversion6/1, Data Type Conversion7/1
  input_voltages_abc/1 -> Data Type Conversion31/1
  Bus Selector1/4 -> [control_dq_abc]  "<control_dq_abc>"
  Bus Selector1/3 -> [switch_pspl]  "<switch_pspl>"
  Bus Selector1/2 -> [sim_mech]  "<simulate_mechanics>"
  Bus Selector1/1 -> [reset]  "<reset_integrators>"
  input_voltages_dq/1 -> Switch2/1
  Data Type Conversion13/1 -> Mux/5  "theta_el"
  Model_Parameter/1 -> Bus Selector1/1
  [reset] -> mechanical_system/1(reset)
  [reset] -> pmsm/1(reset)
  [omega_mech] -> Switch1/3, Switch/3
  [load_torque] -> mechanical_system/6(load_torque)
  Data Type Conversion5/1 -> [load_torque]  "load_torque"
  Data Type Conversion4/1 -> [omega_mech]  "omega_mech"
  pmsm/5(psi_vector) -> Terminator/1
  [np] -> torque_calculation/5(polepairs)
  Mux/1 -> output_general/1
  inputs_general/1 -> Demux/1
  Data Type Conversion26/1 -> Mux/1  "i_d"
  Data Type Conversion11/1 -> Mux/2  "i_q"
  Data Type Conversion15/1 -> Mux/3  "torque"
  Data Type Conversion16/1 -> Mux/4  "omega_mech"
  pmsm/1(I_d) -> torque_calculation/1(I_d), Data Type Conversion26/1, Mux1/1  "i_d"
  pmsm/2(I_q) -> torque_calculation/2(I_q), Data Type Conversion11/1, Mux1/2  "i_q"
  mechanical_system/1(omega_mech) -> Switch1/1, Switch/1
  torque_calculation/1(M_Mi) -> mechanical_system/2(M_Mi), Data Type Conversion15/1
  [sim_mech] -> Switch/2, Switch1/2
  pmsm/4(psi_q) -> torque_calculation/4(psi_q)
  pmsm/3(psi_d) -> torque_calculation/3(psi_d)
  Switch/1 -> pmsm/3(omega_mech)

== system gm_uz_pmsm_model_9ph_vnl/Compare/Assert_output_currents_abc ==
  cosim : Inport
  dut : Inport  Port=2
  AssertEq : Assertion  StopWhenAssertionFail=off
  Compare To Zero : simulink/Logic and Bit Operations/Compare To Zero  relop===  OutDataTypeStr=boolean
  Constant1 : Constant  Value=0  OutDataTypeStr=Inherit: Inherit via back propagation  SampleTime=-1
  Counter : simulink/Sources/Counter Free-Running  NumBits=32  tsamp=-1
  IgnoreCycles : Constant  Value=2  OutDataTypeStr=Inherit: Inherit via back propagation  SampleTime=-1
  RelErrCheck : Subsystem
  Relational Operator : RelationalOperator  Operator=<  OutDataTypeStr=boolean  RndMeth=Nearest
  Switch : Switch  Criteria=u2 ~= 0
  Switch1 : Switch  Criteria=u2 ~= 0
  compare: output_currents_abc : Scope  NumInputPorts=3
  wires:
  IgnoreCycles/1 -> Relational Operator/2
  Counter/1 -> Relational Operator/1
  dut/1 -> Switch/3  "dut ref"
  cosim/1 -> Switch1/3  "cosim"
  Relational Operator/1 -> Switch1/2, Switch/2
  Constant1/1 -> Switch1/1, Switch/1
  Switch/1 -> compare: output_currents_abc/2, RelErrCheck/2(In2)
  Switch1/1 -> compare: output_currents_abc/1, RelErrCheck/1(In1)
  RelErrCheck/1(Out1) -> AssertEq/1, Compare To Zero/1  "err"
  Compare To Zero/1 -> compare: output_currents_abc/3

== system gm_uz_pmsm_model_9ph_vnl/Compare/Assert_output_currents_dq ==
  cosim : Inport
  dut : Inport  Port=2
  AssertEq : Assertion  StopWhenAssertionFail=off
  Compare To Zero : simulink/Logic and Bit Operations/Compare To Zero  relop===  OutDataTypeStr=boolean
  Constant1 : Constant  Value=0  OutDataTypeStr=Inherit: Inherit via back propagation  SampleTime=-1
  Counter : simulink/Sources/Counter Free-Running  NumBits=32  tsamp=-1
  IgnoreCycles : Constant  Value=2  OutDataTypeStr=Inherit: Inherit via back propagation  SampleTime=-1
  RelErrCheck : Subsystem
  Relational Operator : RelationalOperator  Operator=<  OutDataTypeStr=boolean  RndMeth=Nearest
  Switch : Switch  Criteria=u2 ~= 0
  Switch1 : Switch  Criteria=u2 ~= 0
  compare: output_currents_dq : Scope  NumInputPorts=3
  wires:
  IgnoreCycles/1 -> Relational Operator/2
  Counter/1 -> Relational Operator/1
  dut/1 -> Switch/3  "dut ref"
  cosim/1 -> Switch1/3  "cosim"
  Relational Operator/1 -> Switch1/2, Switch/2
  Constant1/1 -> Switch1/1, Switch/1
  Switch/1 -> compare: output_currents_dq/2, RelErrCheck/2(In2)
  Switch1/1 -> compare: output_currents_dq/1, RelErrCheck/1(In1)
  RelErrCheck/1(Out1) -> AssertEq/1, Compare To Zero/1  "err"
  Compare To Zero/1 -> compare: output_currents_dq/3

== system gm_uz_pmsm_model_9ph_vnl/Compare/Assert_output_general ==
  cosim : Inport
  dut : Inport  Port=2
  AssertEq : Assertion  StopWhenAssertionFail=off
  Compare To Zero : simulink/Logic and Bit Operations/Compare To Zero  relop===  OutDataTypeStr=boolean
  Constant1 : Constant  Value=0  OutDataTypeStr=Inherit: Inherit via back propagation  SampleTime=-1
  Counter : simulink/Sources/Counter Free-Running  NumBits=32  tsamp=-1
  IgnoreCycles : Constant  Value=2  OutDataTypeStr=Inherit: Inherit via back propagation  SampleTime=-1
  RelErrCheck : Subsystem
  Relational Operator : RelationalOperator  Operator=<  OutDataTypeStr=boolean  RndMeth=Nearest
  Switch : Switch  Criteria=u2 ~= 0
  Switch1 : Switch  Criteria=u2 ~= 0
  compare: output_general : Scope  NumInputPorts=3
  wires:
  IgnoreCycles/1 -> Relational Operator/2
  Counter/1 -> Relational Operator/1
  dut/1 -> Switch/3  "dut ref"
  cosim/1 -> Switch1/3  "cosim"
  Relational Operator/1 -> Switch1/2, Switch/2
  Constant1/1 -> Switch1/1, Switch/1
  Switch/1 -> compare: output_general/2, RelErrCheck/2(In2)
  Switch1/1 -> compare: output_general/1, RelErrCheck/1(In1)
  RelErrCheck/1(Out1) -> AssertEq/1, Compare To Zero/1  "err"
  Compare To Zero/1 -> compare: output_general/3

== system gm_uz_pmsm_model_9ph_vnl/Compare/Assert_u_abc_pl_out ==
  cosim : Inport
  dut : Inport  Port=2
  AssertEq : Assertion  StopWhenAssertionFail=off
  Compare To Zero : simulink/Logic and Bit Operations/Compare To Zero  relop===  OutDataTypeStr=boolean
  Constant1 : Constant  Value=0  OutDataTypeStr=Inherit: Inherit via back propagation  SampleTime=-1
  Counter : simulink/Sources/Counter Free-Running  NumBits=32  tsamp=-1
  IgnoreCycles : Constant  Value=2  OutDataTypeStr=Inherit: Inherit via back propagation  SampleTime=-1
  Relational Operator : RelationalOperator  Operator=<  OutDataTypeStr=boolean  RndMeth=Nearest
  Relational Operator1 : RelationalOperator  Operator===  OutDataTypeStr=boolean  RndMeth=Nearest
  Switch : Switch  Criteria=u2 ~= 0
  Switch1 : Switch  Criteria=u2 ~= 0
  compare: u_abc_pl_out : Scope  NumInputPorts=3
  wires:
  Compare To Zero/1 -> compare: u_abc_pl_out/3
  Relational Operator1/1 -> Compare To Zero/1, AssertEq/1  "err"
  Switch1/1 -> compare: u_abc_pl_out/1, Relational Operator1/1
  Switch/1 -> compare: u_abc_pl_out/2, Relational Operator1/2
  Constant1/1 -> Switch/1, Switch1/1
  Relational Operator/1 -> Switch/2, Switch1/2
  cosim/1 -> Switch1/3  "cosim"
  dut/1 -> Switch/3  "dut ref"
  Counter/1 -> Relational Operator/1
  IgnoreCycles/1 -> Relational Operator/2

== system gm_uz_pmsm_model_9ph_vnl/Compare/CleanupScopes ==

== system gm_uz_pmsm_model_9ph_vnl/Compare/Enable ==

== system gm_uz_pmsm_model_9ph_vnl/FOC_controller/decoupling ==
  i_d : Inport
  i_q : Inport  Port=2
  omega_m : Inport  Port=3
  Constant1 : Constant  Value=psi_pm  SampleTime=-1
  Gain : Gain  Gain=L_q
  Gain1 : Gain  Gain=L_d
  Gain2 : Gain  Gain=polepair
  Product : Product
  Product1 : Product
  Sum6 : Sum  Inputs=|++
  u_d : Outport
  u_q : Outport  Port=2
  wires:
  Gain/1 -> Product/1
  Gain2/1 -> Product1/2, Product/2
  Product1/1 -> u_q/1
  i_d/1 -> Gain1/1
  Product/1 -> u_d/1
  Gain1/1 -> Sum6/1
  i_q/1 -> Gain/1
  Constant1/1 -> Sum6/2
  Sum6/1 -> Product1/1
  omega_m/1 -> Gain2/1

== system gm_uz_pmsm_model_9ph_vnl/uz_pmsm_model_9ph/Abs ==
  In1 : Inport
  Abs : Abs  SampleTime=1e-08  OutDataTypeStr=double
  Out1 : Outport
  wires:
  Abs/1 -> Out1/1
  In1/1 -> Abs/1

== system gm_uz_pmsm_model_9ph_vnl/uz_pmsm_model_9ph/Add ==
  In1 : Inport
  In2 : Inport  Port=2
  Add : Sum  Inputs=+-  OutDataTypeStr=double  SampleTime=1e-08
  Out1 : Outport
  wires:
  Add/1 -> Out1/1
  In2/1 -> Add/2
  In1/1 -> Add/1

== system gm_uz_pmsm_model_9ph_vnl/uz_pmsm_model_9ph/Add1 ==
  In1 : Inport
  In2 : Inport  Port=2
  Add1 : Sum  Inputs=+-  OutDataTypeStr=double  SampleTime=1e-08
  Out1 : Outport
  wires:
  Add1/1 -> Out1/1
  In2/1 -> Add1/2
  In1/1 -> Add1/1

== system gm_uz_pmsm_model_9ph_vnl/uz_pmsm_model_9ph/Add2 ==
  In1 : Inport
  In2 : Inport  Port=2
  Add2 : Sum  Inputs=+-  OutDataTypeStr=double  SampleTime=1e-08
  Out1 : Outport
  wires:
  Add2/1 -> Out1/1
  In2/1 -> Add2/2
  In1/1 -> Add2/1

== system gm_uz_pmsm_model_9ph_vnl/uz_pmsm_model_9ph/Add3 ==
  In1 : Inport
  In2 : Inport  Port=2
  Add3 : Sum  Inputs=+-  OutDataTypeStr=double  SampleTime=1e-08
  Out1 : Outport
  wires:
  Add3/1 -> Out1/1
  In2/1 -> Add3/2
  In1/1 -> Add3/1

== system gm_uz_pmsm_model_9ph_vnl/uz_pmsm_model_9ph/Add4 ==
  In1 : Inport
  In2 : Inport  Port=2
  Add4 : Sum  Inputs=+-  OutDataTypeStr=double  SampleTime=1e-08
  Out1 : Outport
  wires:
  Add4/1 -> Out1/1
  In2/1 -> Add4/2
  In1/1 -> Add4/1

== system gm_uz_pmsm_model_9ph_vnl/uz_pmsm_model_9ph/Add5 ==
  In1 : Inport
  In2 : Inport  Port=2
  Add5 : Sum  Inputs=+-  OutDataTypeStr=double  SampleTime=1e-08
  Out1 : Outport
  wires:
  Add5/1 -> Out1/1
  In2/1 -> Add5/2
  In1/1 -> Add5/1

== system gm_uz_pmsm_model_9ph_vnl/uz_pmsm_model_9ph/Add6 ==
  In1 : Inport
  In2 : Inport  Port=2
  Add6 : Sum  Inputs=+-  OutDataTypeStr=double  SampleTime=1e-08
  Out1 : Outport
  wires:
  Add6/1 -> Out1/1
  In2/1 -> Add6/2
  In1/1 -> Add6/1

== system gm_uz_pmsm_model_9ph_vnl/uz_pmsm_model_9ph/Cos_to_sincos ==
  In1 : Inport
  Cos_to_sincos : Trigonometry  Operator=sincos  SampleTime=1e-08
  Out1 : Outport
  Out2 : Outport  Port=2
  wires:
  Cos_to_sincos/2 -> Out2/1
  Cos_to_sincos/1 -> Out1/1
  In1/1 -> Cos_to_sincos/1

== system gm_uz_pmsm_model_9ph_vnl/uz_pmsm_model_9ph/Data Type Conversion1 ==
  In1 : Inport
  Data Type Conversion1 : DataTypeConversion  OutDataTypeStr=double  RndMeth=Nearest  SampleTime=1e-08
  Out1 : Outport
  wires:
  Data Type Conversion1/1 -> Out1/1
  In1/1 -> Data Type Conversion1/1

== system gm_uz_pmsm_model_9ph_vnl/uz_pmsm_model_9ph/Data Type Conversion10 ==
  In1 : Inport
  Data Type Conversion10 : DataTypeConversion  OutDataTypeStr=double  RndMeth=Nearest  SampleTime=1e-08
  Out1 : Outport
  wires:
  Data Type Conversion10/1 -> Out1/1
  In1/1 -> Data Type Conversion10/1

== system gm_uz_pmsm_model_9ph_vnl/uz_pmsm_model_9ph/Data Type Conversion11 ==
  In1 : Inport
  Data Type Conversion11 : DataTypeConversion  OutDataTypeStr=single  RndMeth=Nearest  SampleTime=1e-08
  Out1 : Outport
  wires:
  Data Type Conversion11/1 -> Out1/1
  In1/1 -> Data Type Conversion11/1

== system gm_uz_pmsm_model_9ph_vnl/uz_pmsm_model_9ph/Data Type Conversion111 ==
  In1 : Inport
  Data Type Conversion111 : DataTypeConversion  OutDataTypeStr=double  RndMeth=Nearest  SampleTime=1e-08
  Out1 : Outport
  wires:
  Data Type Conversion111/1 -> Out1/1
  In1/1 -> Data Type Conversion111/1
